simulink model "Linear_Model"  (R2023a)
settings: Solver=VariableStepAuto  StartTime=0.0  StopTime=300  RelTol=1e-3
values from neighbouring files (symbols this model uses):
  A = A_long    [Long_State_Controller.m]    (also in sistem_state_space.m = [LinearAll.System(1, 1).A(1:2,1:2) LinearAll.System(1, 1).A()
  B = B_long    [Long_State_Controller.m]
  C = eye(5)    [Long_Linear_System.m]    (also in Long_State_Controller.m; ackerData.m = zeros(1,n))
  D = [0 0; 0 0; 0 0; 0 0; 0 0]    [Long_Linear_System.m]    (also in Long_State_Controller.m)
  Int_cond = [81;0;0;0;0; 0;5.030425; 52.307678; 1070; 0; 0; 295]    [Linear_System.m]
libraries: cstblocks x1, slpidlib x1
settings Model: Creator=berke  LastModifiedBy=berke

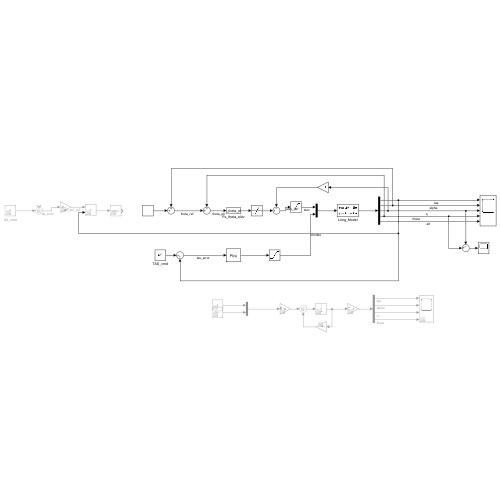
[thumbnail: Simulink's stored preview of the top-level diagram]
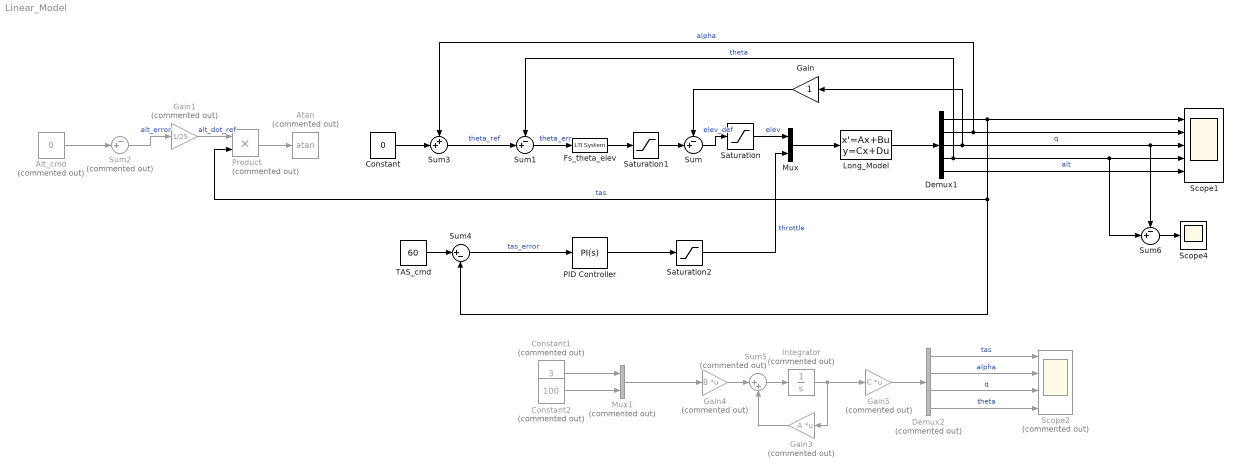
== system Linear_Model ==
  Alt_cmd : Constant  Commented=on  Value=0
  Atan : Trigonometry  Commented=on  Operator=atan
  Constant : Constant  Value=0
  Constant1 : Constant  Commented=on  Value=3
  Constant2 : Constant  Commented=on  Value=100
  Demux1 : Demux  Outputs=5
  Demux2 : Demux  Commented=on
  Fs_theta_elev : cstblocks/LTI System  sys=Fs_theta_elev  IC=[]
  Gain : Gain
  Gain1 : Gain  Commented=on  Gain=1/25
  Gain3 : Gain  Commented=on  Gain=A  Multiplication=Matrix(K*u)
  Gain4 : Gain  Commented=on  Gain=B  Multiplication=Matrix(K*u)
  Gain5 : Gain  Commented=on  Gain=C  Multiplication=Matrix(K*u)
  Integrator : Integrator  Commented=on  InitialCondition=Int_cond
  Long_Model : StateSpace  A=A  B=B  C=C  D=D  InitialCondition=Int_cond
  Mux : Mux  Inputs=2
  Mux1 : Mux  Commented=on  Inputs=2
  PID Controller : slpidlib/PID Controller  Controller=PI  Form=Parallel  TimeDomain=Continuous-time  UseExternalTs=off  SampleTime=-1  IntegratorMethod=Forward Euler  FilterMethod=Forward Euler  ControllerParametersSource=internal  P=537.15  I=0.3104  UseKiTs=off  D=-3.2268  N=100  UseFilter=on  TunerSelectOption=Transfer Function Based (PID Tuner App)  InitialConditionSource=internal  InitialConditionForIntegrator=0  InitialConditionForFilter=0  DifferentiatorICPrevScaledInput=0  ExternalReset=none  TrackingMode=off  Kt=1  LimitOutput=off  SatLimitsSource=internal  UpperSaturationLimit=inf  LowerSaturationLimit=-inf  LinearizeAsGain=on  AntiWindupMode=none  Kb=1  LimitIntegrator=off  UpperIntegratorSaturationLimit=inf  LowerIntegratorSaturationLimit=-inf  POutMin=[]  POutMax=[]  IOutMin=[]  IOutMax=[]  DOutMin=[]  DOutMax=[]  NOutMin=[]  NOutMax=[]  SumOutMin=[]  SumOutMax=[]  SaturationOutMin=[]  SaturationOutMax=[]  PParamMin=[]  PParamMax=[]  IParamMin=[]  IParamMax=[]  DParamMin=[]  DParamMax=[]  NParamMin=[]  NParamMax=[]  KbParamMin=[]  KbParamMax=[]  KtParamMin=[]  KtParamMax=[]  KbOutMin=[]  KbOutMax=[]  KtOutMin=[]  KtOutMax=[]  IntegratorOutMin=[]  IntegratorOutMax=[]  FilterOutMin=[]  FilterOutMax=[]  SumI1OutMin=[]  SumI1OutMax=[]  SumI2OutMin=[]  SumI2OutMax=[]  SumI3OutMin=[]  SumI3OutMax=[]  SumI4OutMin=[]  SumI4OutMax=[]  SumDOutMin=[]  SumDOutMax=[]  DifferentiatorOutMin=[]  DifferentiatorOutMax=[]  FilterDiffOutCoefMin=[]  FilterDiffOutCoefMax=[]  ReciprocalOutMin=[]  ReciprocalOutMax=[]  SumDenOutMin=[]  SumDenOutMax=[]  SumNumOutMin=[]  SumNumOutMax=[]  DivideOutMin=[]  DivideOutMax=[]  UdiffTsProdOutMin=[]  UdiffTsProdOutMax=[]  NTsProdOutMin=[]  NTsProdOutMax=[]  UintegralTsProdOutMin=[]  UintegralTsProdOutMax=[]  UngainTsProdOutMin=[]  UngainTsProdOutMax=[]  ClampingZeroOutDataTypeStr=Inherit: Inherit via back propagation  ClampingZeroOutMin=[]  ClampingZeroOutMax=[]  FilterDenConstantOutDataTypeStr=Inherit: Inherit via back propagation  FilterDenConstantOutMin=[]  FilterDenConstantOutMax=[]  PCopyOutDataTypeStr=Inherit: Inherit via back propagation  PCopyOutMin=[]  PCopyOutMax=[]  NCopyOutDataTypeStr=Inherit: Inherit via back propagation  NCopyOutMin=[]  NCopyOutMax=[]  IntegratorContinuousStateAttributes=''  IntegratorStateMustResolveToSignalObject=off  IntegratorRTWStateStorageClass=Auto  FilterContinuousStateAttributes=''  FilterStateMustResolveToSignalObject=off  FilterRTWStateStorageClass=Auto  ParallelPVariant=InternalParameters  IdealPVariant=Disabled  IVariant=InternalParameters  DVariant=Disabled  IntegratorVariant=Continuous  SatVariant=Disabled  AWVariant=Passthrough  PCopyVariant=Disabled  TRVariant=Disabled  FdbkBlocksVariant=Forward  IdealPFdbkVariant=Disabled  SatFdbkVariant=Disabled  DerivativeFilterVariant=Disabled  NVariant=Disabled  NCopyVariant=Disabled_SignalSpec  FilterICVariant=Disabled  IntegratorICVariant=InternalICs  ExternalResetVariant=Disabled  TRSumVariant=Passthrough  SumFdbkVariant=Disabled  SumVariant=Sum_PI  TsampFilterVariant=InternalTs  TsampNgainVariant=Passthrough  TsampIntegralVariant=Disabled_SignalSpec  ExternalSaturationOutDataTypeStr=Inherit: Same as second input
  Product : Product  Commented=on
  Saturation : Saturate  UpperLimit=30  LowerLimit=-30
  Saturation1 : Saturate  UpperLimit=30  LowerLimit=-30
  Saturation2 : Saturate  UpperLimit=100  LowerLimit=0
  Scope1 : Scope  NumInputPorts=5
  Scope2 : Scope  Commented=on  NumInputPorts=4
  Scope4 : Scope
  Sum : Sum  Inputs=-+|
  Sum1 : Sum  Inputs=-+|
  Sum2 : Sum  Commented=on  Inputs=-+|
  Sum3 : Sum  Inputs=++|
  Sum4 : Sum  Inputs=|+-
  Sum5 : Sum  Commented=on  Inputs=|++
  Sum6 : Sum  Inputs=-+|
  TAS_cmd : Constant  Value=60
  wires:
  Demux1/3 -> Sum6/1, Scope1/3, Gain/1  "q"
  Demux1/2 -> Scope1/2, Sum3/1  "alpha"
  Demux1/4 -> Sum6/2, Scope1/4, Sum1/1  "theta"
  Long_Model/1 -> Demux1/1
  Demux1/1 -> Sum4/2, Product/2, Scope1/1  "tas"
  Sum/1 -> Saturation/1  "elev_def"
  Gain/1 -> Sum/1
  Sum3/1 -> Sum1/2  "theta_ref"
  Alt_cmd/1 -> Sum2/2
  Sum2/1 -> Gain1/1  "alt_error"
  Gain1/1 -> Product/1  "alt_dot_ref"
  Product/1 -> Atan/1
  Saturation1/1 -> Sum/2
  Mux/1 -> Long_Model/1
  Saturation/1 -> Mux/1  "elev"
  Saturation2/1 -> Mux/2  "throttle"
  TAS_cmd/1 -> Sum4/1
  Sum4/1 -> PID Controller/1  "tas_error"
  Sum1/1 -> Fs_theta_elev/1  "theta_err"
  PID Controller/1 -> Saturation2/1
  Fs_theta_elev/1 -> Saturation1/1
  Constant/1 -> Sum3/2
  Constant1/1 -> Mux1/1
  Constant2/1 -> Mux1/2
  Gain4/1 -> Sum5/1
  Gain3/1 -> Sum5/2
  Sum5/1 -> Integrator/1
  Integrator/1 -> Gain5/1, Gain3/1
  Mux1/1 -> Gain4/1
  Gain5/1 -> Demux2/1
  Demux2/1 -> Scope2/1  "tas"
  Demux2/2 -> Scope2/2  "alpha"
  Demux2/3 -> Scope2/3  "q"
  Demux2/4 -> Scope2/4  "theta"
  Demux1/5 -> Scope1/5  "alt"
  Sum6/1 -> Scope4/1
